simulink model "ContinuosBuck_Offine_Control4"  (R2025a)
settings: Solver=VariableStepAuto  StartTime=0.0  StopTime=SimTime  RelTol=RelativeTolerance
undefined symbols (not defined in the file or in its folder): C_buck, Iout_buck, L_buck, R, R1, R2, R3, t1, t2, t2prima, t3, Tsim, Tsw, Vg, Vout_buck
libraries: slpidlib x3, spsPWMGeneratorDCDCLib x1
settings Model: Creator=Andres  LastModifiedBy=nelso
settings DataIOCC: SaveFormat=StructureWithTime  ReturnWorkspaceOutputs=off  SignalLoggingName=ResultCont

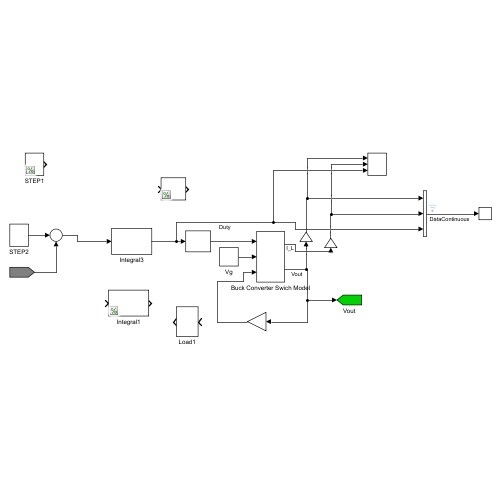
[thumbnail: Simulink's stored preview of the top-level diagram]
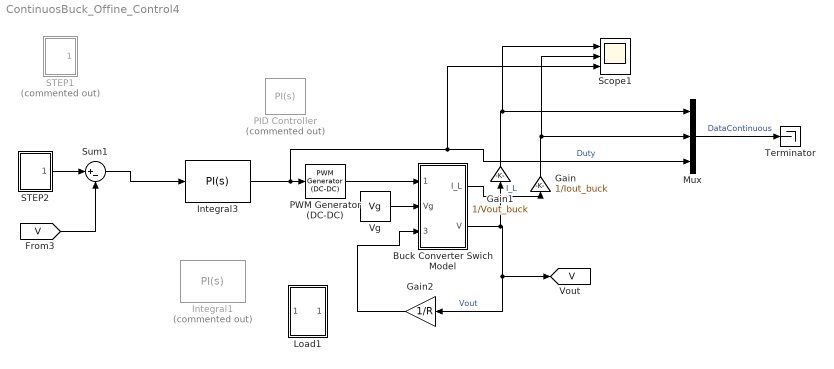
== system ContinuosBuck_Offine_Control4 ==
  Buck Converter Swich Model : Subsystem
      mask Display: image('$imagefile'); % Use "Edit Image" on toolstrip to change.
  Gain : Gain  Gain=1/Iout_buck
  Gain1 : Gain  Gain=1/Vout_buck
  Gain2 : Gain  Gain=1/R
  Integral1 : slpidlib/PID Controller  Commented=on  Controller=PI  Form=Parallel  TimeDomain=Continuous-time  UseExternalTs=on  SampleTime=Tsw  IntegratorMethod=Trapezoidal  FilterMethod=Forward Euler  ControllerParametersSource=internal  P=0.000518134045814252  I=108.332907969673  UseKiTs=off  D=1.78707996704397e-06  UseExternalDerivativeSource=off  N=1  UseFilter=on  TunerSelectOption=Transfer Function Based (PID Tuner App)  InitialConditionSource=internal  InitialConditionForIntegrator=0  InitialConditionForFilter=0  DifferentiatorICPrevScaledInput=0  ExternalReset=none  IgnoreLimit=on  TrackingMode=off  Kt=1  LimitOutput=on  SatLimitsSource=internal  UpperSaturationLimit=0.98  LowerSaturationLimit=0  LinearizeAsGain=on  AntiWindupMode=clamping  Kb=1  LimitIntegrator=off  UpperIntegratorSaturationLimit=inf  LowerIntegratorSaturationLimit=-inf  POutMin=[]  POutMax=[]  IOutMin=[]  IOutMax=[]  DOutMin=[]  DOutMax=[]  NOutMin=[]  NOutMax=[]  SumOutMin=[]  SumOutMax=[]  SaturationOutMin=[]  SaturationOutMax=[]  PParamMin=[]  PParamMax=[]  IParamMin=[]  IParamMax=[]  DParamMin=[]  DParamMax=[]  NParamMin=[]  NParamMax=[]  KbParamMin=[]  KbParamMax=[]  KtParamMin=[]  KtParamMax=[]  KbOutMin=[]  KbOutMax=[]  KtOutMin=[]  KtOutMax=[]  IntegratorOutMin=[]  IntegratorOutMax=[]  FilterOutMin=[]  FilterOutMax=[]  SumI1OutMin=[]  SumI1OutMax=[]  SumI2OutMin=[]  SumI2OutMax=[]  SumI3OutMin=[]  SumI3OutMax=[]  SumI4OutMin=[]  SumI4OutMax=[]  SumDOutMin=[]  SumDOutMax=[]  DifferentiatorOutMin=[]  DifferentiatorOutMax=[]  FilterDiffOutCoefMin=[]  FilterDiffOutCoefMax=[]  ReciprocalOutMin=[]  ReciprocalOutMax=[]  SumDenOutMin=[]  SumDenOutMax=[]  SumNumOutMin=[]  SumNumOutMax=[]  DivideOutMin=[]  DivideOutMax=[]  UdiffTsProdOutMin=[]  UdiffTsProdOutMax=[]  NTsProdOutMin=[]  NTsProdOutMax=[]  UintegralTsProdOutMin=[]  UintegralTsProdOutMax=[]  UngainTsProdOutMin=[]  UngainTsProdOutMax=[]  ClampingZeroOutDataTypeStr=Inherit: Inherit via back propagation  ClampingZeroOutMin=[]  ClampingZeroOutMax=[]  FilterDenConstantOutDataTypeStr=Inherit: Inherit via back propagation  FilterDenConstantOutMin=[]  FilterDenConstantOutMax=[]  PCopyOutDataTypeStr=Inherit: Inherit via back propagation  PCopyOutMin=[]  PCopyOutMax=[]  NCopyOutDataTypeStr=Inherit: Inherit via back propagation  NCopyOutMin=[]  NCopyOutMax=[]  IntegratorContinuousStateAttributes=''  IntegratorStateMustResolveToSignalObject=off  IntegratorRTWStateStorageClass=Auto  FilterContinuousStateAttributes=''  FilterStateMustResolveToSignalObject=off  FilterRTWStateStorageClass=Auto  ParallelPVariant=InternalParameters  IdealPVariant=Disabled  IVariant=InternalParameters  DVariant=Disabled  IntegratorVariant=Continuous  SatVariant=Enabled  AWVariant=ContClampingParallel  PCopyVariant=Disabled  TRVariant=Disabled  FdbkBlocksVariant=Forward  IdealPFdbkVariant=Disabled  SatFdbkVariant=Disabled  DerivativeFilterVariant=Disabled  NVariant=Disabled  NCopyVariant=Disabled_SignalSpec  FilterICVariant=Disabled  IntegratorICVariant=InternalICs  ExternalResetVariant=Disabled  TRSumVariant=Passthrough  SumFdbkVariant=Disabled  SumVariant=Sum_PI  TsampFilterVariant=InternalTs  TsampNgainVariant=Passthrough  TsampIntegralVariant=Disabled_SignalSpec  ExternalSaturationOutDataTypeStr=Inherit: Same as second input  DerivativeSourceVariant=Disabled  PreIntVariant=InternalPreInt
  Integral3 : slpidlib/PID Controller  Controller=PI  Form=Parallel  TimeDomain=Continuous-time  UseExternalTs=on  SampleTime=Tsw  IntegratorMethod=Trapezoidal  FilterMethod=Forward Euler  ControllerParametersSource=internal  P=0  I=63.9226  UseKiTs=off  D=1.78707996704397e-06  UseExternalDerivativeSource=off  N=1  UseFilter=on  TunerSelectOption=Transfer Function Based (PID Tuner App)  InitialConditionSource=internal  InitialConditionForIntegrator=0  InitialConditionForFilter=0  DifferentiatorICPrevScaledInput=0  ExternalReset=none  IgnoreLimit=on  TrackingMode=off  Kt=1  LimitOutput=on  SatLimitsSource=internal  UpperSaturationLimit=0.98  LowerSaturationLimit=0  LinearizeAsGain=on  AntiWindupMode=clamping  Kb=1  LimitIntegrator=off  UpperIntegratorSaturationLimit=inf  LowerIntegratorSaturationLimit=-inf  POutMin=[]  POutMax=[]  IOutMin=[]  IOutMax=[]  DOutMin=[]  DOutMax=[]  NOutMin=[]  NOutMax=[]  SumOutMin=[]  SumOutMax=[]  SaturationOutMin=[]  SaturationOutMax=[]  PParamMin=[]  PParamMax=[]  IParamMin=[]  IParamMax=[]  DParamMin=[]  DParamMax=[]  NParamMin=[]  NParamMax=[]  KbParamMin=[]  KbParamMax=[]  KtParamMin=[]  KtParamMax=[]  KbOutMin=[]  KbOutMax=[]  KtOutMin=[]  KtOutMax=[]  IntegratorOutMin=[]  IntegratorOutMax=[]  FilterOutMin=[]  FilterOutMax=[]  SumI1OutMin=[]  SumI1OutMax=[]  SumI2OutMin=[]  SumI2OutMax=[]  SumI3OutMin=[]  SumI3OutMax=[]  SumI4OutMin=[]  SumI4OutMax=[]  SumDOutMin=[]  SumDOutMax=[]  DifferentiatorOutMin=[]  DifferentiatorOutMax=[]  FilterDiffOutCoefMin=[]  FilterDiffOutCoefMax=[]  ReciprocalOutMin=[]  ReciprocalOutMax=[]  SumDenOutMin=[]  SumDenOutMax=[]  SumNumOutMin=[]  SumNumOutMax=[]  DivideOutMin=[]  DivideOutMax=[]  UdiffTsProdOutMin=[]  UdiffTsProdOutMax=[]  NTsProdOutMin=[]  NTsProdOutMax=[]  UintegralTsProdOutMin=[]  UintegralTsProdOutMax=[]  UngainTsProdOutMin=[]  UngainTsProdOutMax=[]  ClampingZeroOutDataTypeStr=Inherit: Inherit via back propagation  ClampingZeroOutMin=[]  ClampingZeroOutMax=[]  FilterDenConstantOutDataTypeStr=Inherit: Inherit via back propagation  FilterDenConstantOutMin=[]  FilterDenConstantOutMax=[]  PCopyOutDataTypeStr=Inherit: Inherit via back propagation  PCopyOutMin=[]  PCopyOutMax=[]  NCopyOutDataTypeStr=Inherit: Inherit via back propagation  NCopyOutMin=[]  NCopyOutMax=[]  IntegratorContinuousStateAttributes=''  IntegratorStateMustResolveToSignalObject=off  IntegratorRTWStateStorageClass=Auto  FilterContinuousStateAttributes=''  FilterStateMustResolveToSignalObject=off  FilterRTWStateStorageClass=Auto  ParallelPVariant=InternalParameters  IdealPVariant=Disabled  IVariant=InternalParameters  DVariant=Disabled  IntegratorVariant=Continuous  SatVariant=Enabled  AWVariant=ContClampingParallel  PCopyVariant=Disabled  TRVariant=Disabled  FdbkBlocksVariant=Forward  IdealPFdbkVariant=Disabled  SatFdbkVariant=Disabled  DerivativeFilterVariant=Disabled  NVariant=Disabled  NCopyVariant=Disabled_SignalSpec  FilterICVariant=Disabled  IntegratorICVariant=InternalICs  ExternalResetVariant=Disabled  TRSumVariant=Passthrough  SumFdbkVariant=Disabled  SumVariant=Sum_PI  TsampFilterVariant=InternalTs  TsampNgainVariant=Passthrough  TsampIntegralVariant=Disabled_SignalSpec  ExternalSaturationOutDataTypeStr=Inherit: Same as second input  DerivativeSourceVariant=Disabled  PreIntVariant=InternalPreInt
  Load1 : Subsystem
  Mux : Mux  Inputs=3
  PID Controller : slpidlib/PID Controller  Commented=on  Controller=PI  Form=Parallel  TimeDomain=Continuous-time  UseExternalTs=off  SampleTime=-1  IntegratorMethod=Forward Euler  FilterMethod=Forward Euler  ControllerParametersSource=internal  P=0.0995683460340593  I=172.683701506663  UseKiTs=off  D=0  UseExternalDerivativeSource=off  N=100  UseFilter=on  TunerSelectOption=Transfer Function Based (PID Tuner App)  InitialConditionSource=internal  InitialConditionForIntegrator=0  InitialConditionForFilter=0  DifferentiatorICPrevScaledInput=0  ExternalReset=none  TrackingMode=off  Kt=1  LimitOutput=off  SatLimitsSource=internal  UpperSaturationLimit=inf  LowerSaturationLimit=-inf  LinearizeAsGain=on  AntiWindupMode=none  Kb=1  LimitIntegrator=off  UpperIntegratorSaturationLimit=inf  LowerIntegratorSaturationLimit=-inf  POutMin=[]  POutMax=[]  IOutMin=[]  IOutMax=[]  DOutMin=[]  DOutMax=[]  NOutMin=[]  NOutMax=[]  SumOutMin=[]  SumOutMax=[]  SaturationOutMin=[]  SaturationOutMax=[]  PParamMin=[]  PParamMax=[]  IParamMin=[]  IParamMax=[]  DParamMin=[]  DParamMax=[]  NParamMin=[]  NParamMax=[]  KbParamMin=[]  KbParamMax=[]  KtParamMin=[]  KtParamMax=[]  KbOutMin=[]  KbOutMax=[]  KtOutMin=[]  KtOutMax=[]  IntegratorOutMin=[]  IntegratorOutMax=[]  FilterOutMin=[]  FilterOutMax=[]  SumI1OutMin=[]  SumI1OutMax=[]  SumI2OutMin=[]  SumI2OutMax=[]  SumI3OutMin=[]  SumI3OutMax=[]  SumI4OutMin=[]  SumI4OutMax=[]  SumDOutMin=[]  SumDOutMax=[]  DifferentiatorOutMin=[]  DifferentiatorOutMax=[]  FilterDiffOutCoefMin=[]  FilterDiffOutCoefMax=[]  ReciprocalOutMin=[]  ReciprocalOutMax=[]  SumDenOutMin=[]  SumDenOutMax=[]  SumNumOutMin=[]  SumNumOutMax=[]  DivideOutMin=[]  DivideOutMax=[]  UdiffTsProdOutMin=[]  UdiffTsProdOutMax=[]  NTsProdOutMin=[]  NTsProdOutMax=[]  UintegralTsProdOutMin=[]  UintegralTsProdOutMax=[]  UngainTsProdOutMin=[]  UngainTsProdOutMax=[]  ClampingZeroOutDataTypeStr=Inherit: Inherit via back propagation  ClampingZeroOutMin=[]  ClampingZeroOutMax=[]  FilterDenConstantOutDataTypeStr=Inherit: Inherit via back propagation  FilterDenConstantOutMin=[]  FilterDenConstantOutMax=[]  PCopyOutDataTypeStr=Inherit: Inherit via back propagation  PCopyOutMin=[]  PCopyOutMax=[]  NCopyOutDataTypeStr=Inherit: Inherit via back propagation  NCopyOutMin=[]  NCopyOutMax=[]  IntegratorContinuousStateAttributes=''  IntegratorStateMustResolveToSignalObject=off  IntegratorRTWStateStorageClass=Auto  FilterContinuousStateAttributes=''  FilterStateMustResolveToSignalObject=off  FilterRTWStateStorageClass=Auto  ParallelPVariant=InternalParameters  IdealPVariant=Disabled  IVariant=InternalParameters  DVariant=Disabled  IntegratorVariant=Continuous  SatVariant=Disabled  AWVariant=Passthrough  PCopyVariant=Disabled  TRVariant=Disabled  FdbkBlocksVariant=Forward  IdealPFdbkVariant=Disabled  SatFdbkVariant=Disabled  DerivativeFilterVariant=Disabled  NVariant=Disabled  NCopyVariant=Disabled_SignalSpec  FilterICVariant=Disabled  IntegratorICVariant=InternalICs  ExternalResetVariant=Disabled  TRSumVariant=Passthrough  SumFdbkVariant=Disabled  SumVariant=Sum_PI  TsampFilterVariant=InternalTs  TsampNgainVariant=Passthrough  TsampIntegralVariant=Disabled_SignalSpec  ExternalSaturationOutDataTypeStr=Inherit: Same as second input  DerivativeSourceVariant=Disabled  PreIntVariant=InternalPreInt
  PWM Generator (DC-DC) : spsPWMGeneratorDCDCLib/PWM Generator (DC-DC)  Fsw=f_sw  Ts=0
  STEP1 : Subsystem  Commented=on
  STEP2 : Subsystem
  Scope1 : Scope  NumInputPorts=3
      settings: ActiveDisplayYMinimum=-0.30543358970666512  ActiveDisplayYMaximum=2.7489023073599865  YLabel=Voltage (V)
  Sum1 : Sum  Inputs=|+-
  Terminator : Terminator
  Vg : Constant  Value=Vg  SampleTime=-1
  tag scope: V=global
  wires:
  Integral3/1 -> Scope1/3, Mux/3, PWM Generator (DC-DC)/1  "Duty"
  STEP2/1(STEP) -> Sum1/1
  [V] -> Sum1/2
  Sum1/1 -> Integral3/1
  Gain2/1 -> Buck Converter Swich Model/3(I_load)
  Buck Converter Swich Model/1(I_L) -> Gain/1  "I_L"
  Buck Converter Swich Model/2(V) -> Gain1/1, Gain2/1, [V]  "Vout"
  PWM Generator (DC-DC)/1 -> Buck Converter Swich Model/1(PWM)
  Vg/1 -> Buck Converter Swich Model/2(Vg)
  Mux/1 -> Terminator/1  "DataContinuous"
  Gain/1 -> Mux/2, Scope1/2
  Gain1/1 -> Mux/1, Scope1/1

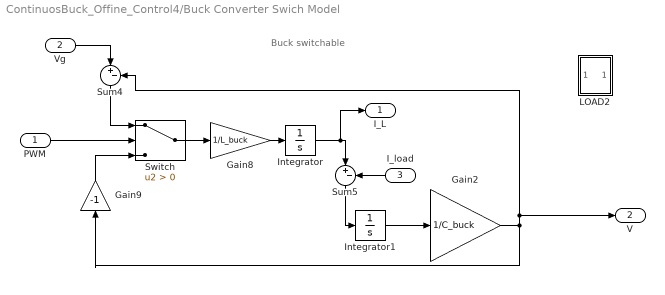
== system ContinuosBuck_Offine_Control4/Buck Converter Swich Model ==
  note: Buck switchable
  PWM : Inport
  Vg : Inport  Port=2
  I_load : Inport  Port=3
  Gain2 : Gain  Gain=1/C_buck
  Gain8 : Gain  Gain=1/L_buck
  Gain9 : Gain  Gain=-1
  Integrator : Integrator  LimitOutput=on  LowerSaturationLimit=0
  Integrator1 : Integrator
  LOAD2 : Subsystem
  Sum4 : Sum  Inputs=|+-
  Sum5 : Sum  Inputs=|+-
  Switch : Switch  Criteria=u2 > Threshold  SaturateOnIntegerOverflow=off  InputSameDT=off
  I_L : Outport
  V : Outport  Port=2
  wires:
  Gain9/1 -> Switch/3
  Switch/1 -> Gain8/1
  Sum4/1 -> Switch/1
  Gain8/1 -> Integrator/1
  Sum5/1 -> Integrator1/1
  Integrator/1 -> I_L/1, Sum5/1
  Vg/1 -> Sum4/1
  I_load/1 -> Sum5/2
  PWM/1 -> Switch/2
  Gain2/1 -> Gain9/1, V/1, Sum4/2
  Integrator1/1 -> Gain2/1

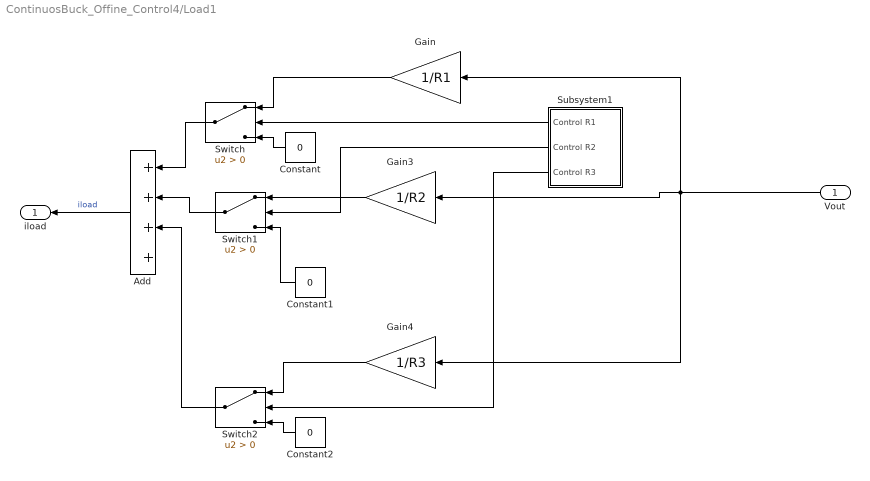
== system ContinuosBuck_Offine_Control4/Load1 ==
  Vout : Inport
  Add : Sum  Inputs=++++
  Constant : Constant  Value=0
  Constant1 : Constant  Value=0
  Constant2 : Constant  Value=0
  Gain : Gain  Gain=1/R1
  Gain3 : Gain  Gain=1/R2
  Gain4 : Gain  Gain=1/R3
  Subsystem1 : Subsystem
  Switch : Switch  Criteria=u2 > Threshold  SaturateOnIntegerOverflow=off  InputSameDT=off
  Switch1 : Switch  Criteria=u2 > Threshold  SaturateOnIntegerOverflow=off  InputSameDT=off
  Switch2 : Switch  Criteria=u2 > Threshold  SaturateOnIntegerOverflow=off  InputSameDT=off
  iload : Outport
  wires:
  Add/1 -> iload/1  "iload"
  Gain3/1 -> Switch1/1
  Constant/1 -> Switch/3
  Subsystem1/3(Control R3) -> Switch2/2
  Switch1/1 -> Add/2
  Constant2/1 -> Switch2/3
  Switch/1 -> Add/1
  Vout/1 -> Gain3/1, Gain/1, Gain4/1
  Subsystem1/1(Control R1) -> Switch/2
  Subsystem1/2(Control R2) -> Switch1/2
  Gain/1 -> Switch/1
  Gain4/1 -> Switch2/1
  Switch2/1 -> Add/3
  Constant1/1 -> Switch1/3

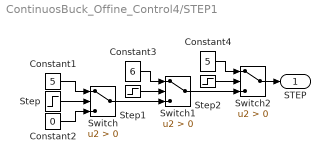
== system ContinuosBuck_Offine_Control4/STEP1 ==
  Constant1 : Constant  Value=5
  Constant2 : Constant  Value=0
  Constant3 : Constant  Value=6
  Constant4 : Constant  Value=5
  Step : Step  Time=0.01
  Step1 : Step  Time=0.05
  Step2 : Step  Time=0.1
  Switch : Switch  Criteria=u2 > Threshold  SaturateOnIntegerOverflow=off  InputSameDT=off
  Switch1 : Switch  Criteria=u2 > Threshold  SaturateOnIntegerOverflow=off  InputSameDT=off
  Switch2 : Switch  Criteria=u2 > Threshold  SaturateOnIntegerOverflow=off  InputSameDT=off
  STEP : Outport
  wires:
  Switch2/1 -> STEP/1
  Constant4/1 -> Switch2/1
  Step2/1 -> Switch2/2
  Switch1/1 -> Switch2/3
  Constant2/1 -> Switch/3
  Step1/1 -> Switch1/2
  Switch/1 -> Switch1/3
  Constant1/1 -> Switch/1
  Constant3/1 -> Switch1/1
  Step/1 -> Switch/2

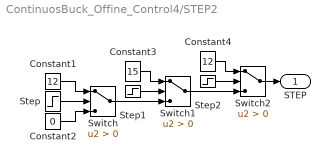
== system ContinuosBuck_Offine_Control4/STEP2 ==
  Constant1 : Constant  Value=12  SampleTime=-1
  Constant2 : Constant  Value=0  SampleTime=-1
  Constant3 : Constant  Value=15  SampleTime=-1
  Constant4 : Constant  Value=12  SampleTime=-1
  Step : Step  Time=0.01
  Step1 : Step  Time=0.03
  Step2 : Step  Time=0.055
  Switch : Switch  Criteria=u2 > Threshold  SaturateOnIntegerOverflow=off  InputSameDT=off
  Switch1 : Switch  Criteria=u2 > Threshold  SaturateOnIntegerOverflow=off  InputSameDT=off
  Switch2 : Switch  Criteria=u2 > Threshold  SaturateOnIntegerOverflow=off  InputSameDT=off
  STEP : Outport
  wires:
  Step/1 -> Switch/2
  Constant3/1 -> Switch1/1
  Constant1/1 -> Switch/1
  Switch/1 -> Switch1/3
  Step1/1 -> Switch1/2
  Constant2/1 -> Switch/3
  Switch1/1 -> Switch2/3
  Step2/1 -> Switch2/2
  Constant4/1 -> Switch2/1
  Switch2/1 -> STEP/1

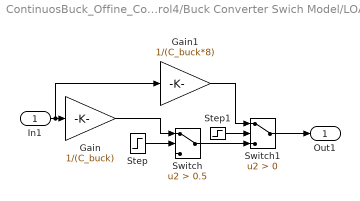
== system ContinuosBuck_Offine_Control4/Buck Converter Swich Model/LOAD2 ==
  In1 : Inport
  Gain : Gain  Gain=1/(C_buck)
  Gain1 : Gain  Gain=1/(C_buck*8)
  Step : Step  Time=0  SampleTime=Tsim
  Step1 : Step  Time=0.07  SampleTime=Tsim
  Switch : Switch  Criteria=u2 > Threshold  Threshold=0.5  SaturateOnIntegerOverflow=off  InputSameDT=off
  Switch1 : Switch  Criteria=u2 > Threshold  SaturateOnIntegerOverflow=off  InputSameDT=off
  Out1 : Outport
  wires:
  Gain1/1 -> Switch1/1
  Step/1 -> Switch/2
  Switch/1 -> Switch1/3
  Step1/1 -> Switch1/2
  Switch1/1 -> Out1/1
  In1/1 -> Gain/1, Gain1/1
  Gain/1 -> Switch/1

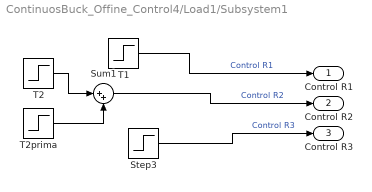
== system ContinuosBuck_Offine_Control4/Load1/Subsystem1 ==
  Step3 : Step  Time=t3  SampleTime=0
  Sum1 : Sum  Inputs=|++
  T1 : Step  Time=t1  Before=1  After=0  SampleTime=0
  T2 : Step  Time=t2  SampleTime=0
  T2prima : Step  Time=t2prima  After=-1  SampleTime=0
  Control R1 : Outport
  Control R2 : Outport  Port=2
  Control R3 : Outport  Port=3
  wires:
  Sum1/1 -> Control R2/1  "Control R2"
  T1/1 -> Control R1/1  "Control R1"
  T2prima/1 -> Sum1/2
  T2/1 -> Sum1/1
  Step3/1 -> Control R3/1  "Control R3"
